simulink model "parity_bit_experiment"  (R2018b)
settings: Solver=VariableStepAuto  StartTime=0.0  StopTime=10.0  RelTol=1e-3
libraries: commrandsrc3 x1, simulink x1
settings Model: Creator=inha  LastModifiedBy=inha

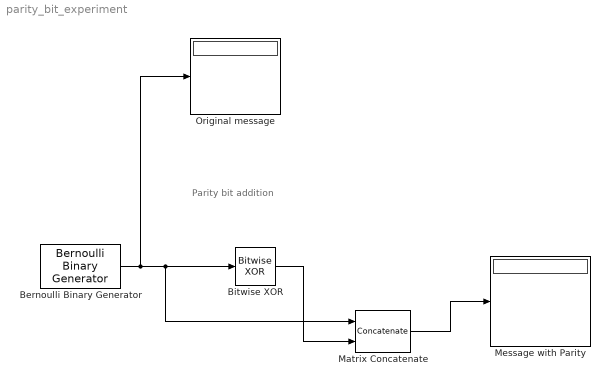
== system parity_bit_experiment ==
  note: Parity bit addition
  Bernoulli Binary Generator : commrandsrc3/Bernoulli Binary Generator  ProbabilityOfZero=0.5  SeedSource=Auto  Seed=0  SampleTime=1  SamplesPerFrame=4  OutputDataType=uint8  SimulateUsing=Interpreted execution
  Bitwise XOR : simulink/Logic and Bit Operations/Bitwise Operator  logicop=XOR  UseBitMask=off  BitMask=bin2dec('11011001')  BitMaskRealWorld=Stored Integer
  Matrix Concatenate : Concatenate  Mode=Multidimensional array
  Message with Parity : Display
  Original message : Display
  wires:
  Bitwise XOR/1 -> Matrix Concatenate/2
  Bernoulli Binary Generator/1 -> Original message/1, Matrix Concatenate/1, Bitwise XOR/1
  Matrix Concatenate/1 -> Message with Parity/1
